simulink model "DFADAS2_SenFus_v1_201204RC_training_210115"  (R2018b)
settings: Solver=FixedStepDiscrete  StartTime=0.0  StopTime=inf  FixedStep=0.002  RelTol=1e-3  EnableMultiTasking=on
PreLoadFcn:
  | RTWConfigurationCB('preloadfcn', bdroot);
libraries: canmsglib x108, simulink x48, canfdmsglib x12
(part 13 of 28)

== system DFADAS2_SenFus_v1_201204RC_training_210115/Signal Input (Input)/Signal Input (50ms) (Input50)/Front Left Radar(S2) Objects Information (FLRdr)/S0 Data Frame Read/Subsystem ==
  Bus Creator : BusCreator  Inputs=10
  M0ObjInfo : Subsystem  TreatAsAtomicUnit=on
  M1ObjInfo1 : Subsystem  TreatAsAtomicUnit=on
  M2ObjInfo : Subsystem  TreatAsAtomicUnit=on
  M3ObjInfo : Subsystem  TreatAsAtomicUnit=on
  M4ObjInfo1 : Subsystem  TreatAsAtomicUnit=on
  RLRdrObjInfo : Outport
  wires:
  Bus Creator/1 -> RLRdrObjInfo/1  "RLRdrObjInfo"
  M1ObjInfo1/1(M10ObjInfo) -> Bus Creator/3  "M10ObjInfo"
  M3ObjInfo/1(M30ObjInfo) -> Bus Creator/7  "M30ObjInfo"
  M4ObjInfo1/1(M40ObjInfo) -> Bus Creator/9  "M40ObjInfo"
  M0ObjInfo/1(M00ObjInfo) -> Bus Creator/1  "M00ObjInfo"
  M2ObjInfo/1(M20ObjInfo) -> Bus Creator/5  "M20ObjInfo"
  M3ObjInfo/2(M31ObjInfo) -> Bus Creator/8  "M31ObjInfo"
  M0ObjInfo/2(M01ObjInfo) -> Bus Creator/2  "M01ObjInfo"
  M1ObjInfo1/2(M11ObjInfo) -> Bus Creator/4  "M11ObjInfo"
  M2ObjInfo/2(M21ObjInfo) -> Bus Creator/6  "M21ObjInfo"
  M4ObjInfo1/2(M41ObjInfo) -> Bus Creator/10  "M41ObjInfo"

== system DFADAS2_SenFus_v1_201204RC_training_210115/Signal Input (Input)/Signal Input (50ms) (Input50)/Front Left Radar(S2) Objects Information (FLRdr)/S0 Data Frame Read/VsblMnmt ==
  note: 虚拟帧的数据帧与Trailer帧的可见性管理逻辑
      | ——包括了对VFCnt回卷的考虑
  HFVFCnt : Inport
  LocVFCnt : Inport  Port=2
  Add : Sum  Inputs=+-
  Constant : Constant  Value=100
  Logical Operator : Logic  Operator=OR  AllPortsSameDT=off  OutDataTypeStr=boolean
  Relational Operator1 : RelationalOperator  OutDataTypeStr=boolean  RndMeth=Simplest
  Relational Operator2 : RelationalOperator  OutDataTypeStr=boolean  RndMeth=Simplest
  EnFlg : Outport
  wires:
  Add/1 -> Relational Operator2/1
  Constant/1 -> Relational Operator2/2
  Logical Operator/1 -> EnFlg/1
  Relational Operator2/1 -> Logical Operator/2
  HFVFCnt/1 -> Relational Operator1/1, Add/2
  Relational Operator1/1 -> Logical Operator/1
  LocVFCnt/1 -> Relational Operator1/2, Add/1

== system DFADAS2_SenFus_v1_201204RC_training_210115/Signal Input (Input)/Signal Input (50ms) (Input50)/Front Left Radar(S2) Objects Information (FLRdr)/S0 Header Frame Read/Enabled Subsystem ==
  note: Reset
  Msg : Inport
  Enable : EnablePort  StatesWhenEnabling=reset
  Bus Creator : BusCreator  Inputs=4
  CAN FD Unpack1 : canfdmsglib/CAN FD Unpack  CANdbFile=C:\Users\ThinkPad\Desktop\200529-海拉角雷达DBC\PR53671_DFPV_D53_HWA_SDE_F-SRR_CANFD_DF RESEARCH.dbc  MsgList=Object_Header_S2  MsgName=Object_Header_S2  ProtocolMode=CAN FD  MsgIDType=Standard (11-bit identifier)  MsgIdentifier=854  MsgLength=20  SignalInfo=NumberOfObjects_S2$67$5$1$2$1$0$1$0$0$30$#StateInfo_S2$0$3$1$2$1$0$1$0$0$7$#gPTPTimeStampOfData_HIGH_S2$35$32$1$2$1$0$1$0$0$4294967295$#gPTPTimeStampOfData_LOW_S2$3$32$1$2$1$0$1$0$0$4294967295$#  NSignals=4  IDPort=off  TimestampPort=off  ErrorPort=off  RemotePort=off  LengthPort=off  StatusPort=off  BRSPort=off  ESIPort=off  DLCPort=off  StartBits=str2num('[int32(67);int32(0);int32(35);int32(3)]')  SignalSizes=str2num('[int32(5);int32(3);int32(32);int32(32)]')  ByteOrders=str2num('[int32(1);int32(1);int32(1);int32(1)]')  DataTypes=str2num('[int32(2);int32(2);int32(2);int32(2)]')  MultiplexTypes=str2num('[int32(1);int32(1);int32(1);int32(1)]')  MultiplexValues=str2num('[double(0);double(0);double(0);double(0)]')  Factors=str2num('[double(1);double(1);double(1);double(1)]')  Offsets=str2num('[double(0);double(0);double(0);double(0)]')  Minimums=str2num('[double(0);double(0);double(0);double(0)]')  Maximums=str2num('[double(30);double(7);double(4294967295);double(4294967295)]')  ApplyMinMax=off
      settings: SourceProductName=Simulink Real-Time  DataFormat=manually specified signals
  Sigs : Outport
  wires:
  Msg/1 -> CAN FD Unpack1/1
  Bus Creator/1 -> Sigs/1  "FLRdr_bsCmnInfo"
  CAN FD Unpack1/1 -> Bus Creator/1  "NumberOfObjects_S2"
  CAN FD Unpack1/2 -> Bus Creator/2  "StateInfo_S2"
  CAN FD Unpack1/3 -> Bus Creator/3  "gPTPTimeStampOfData_LOW_S2"
  CAN FD Unpack1/4 -> Bus Creator/4  "gPTPTimeStampOfData_HIGH_S2"

== system DFADAS2_SenFus_v1_201204RC_training_210115/Signal Input (Input)/Signal Input (50ms) (Input50)/Front Left Radar(S2) Objects Information (FLRdr)/S0 Trailer Frame Read/VsblMnmt ==
  note: 虚拟帧的数据帧与Trailer帧的可见性管理逻辑
      | ——包括了对VFCnt回卷的考虑
  HFVFCnt : Inport
  LocVFCnt : Inport  Port=2
  Add : Sum  Inputs=+-
  Constant : Constant  Value=100
  Logical Operator : Logic  Operator=OR  AllPortsSameDT=off  OutDataTypeStr=boolean
  Relational Operator1 : RelationalOperator  OutDataTypeStr=boolean  RndMeth=Simplest
  Relational Operator2 : RelationalOperator  OutDataTypeStr=boolean  RndMeth=Simplest
  EnFlg : Outport
  wires:
  Add/1 -> Relational Operator2/1
  Constant/1 -> Relational Operator2/2
  Logical Operator/1 -> EnFlg/1
  Relational Operator2/1 -> Logical Operator/2
  HFVFCnt/1 -> Relational Operator1/1, Add/2
  Relational Operator1/1 -> Logical Operator/1
  LocVFCnt/1 -> Relational Operator1/2, Add/1

== system DFADAS2_SenFus_v1_201204RC_training_210115/Signal Input (Input)/Signal Input (50ms) (Input50)/Front Right Radar(S3) Objects Information (FRRdr)/S0 Data Frame Read/Enabled Subsystem ==
  note: Reset
  RemainderCnt : Inport
  Msg : Inport  Port=2
  obj_num : Inport  Port=3
  Enable : EnablePort  StatesWhenEnabling=reset
  Bus Creator : BusCreator  Inputs=10
  M0ObjInfo : Subsystem  TreatAsAtomicUnit=on
  M1ObjInfo1 : Subsystem  TreatAsAtomicUnit=on
  M2ObjInfo : Subsystem  TreatAsAtomicUnit=on
  M3ObjInfo : Subsystem  TreatAsAtomicUnit=on
  M4ObjInfo1 : Subsystem  TreatAsAtomicUnit=on
  Unpack : Subsystem
  RLRdrObjInfo : Outport
  wires:
  Msg/1 -> Unpack/1(Msg)
  Unpack/1(MsgOut) -> M0ObjInfo/1(msg), M4ObjInfo1/1(msg), M3ObjInfo/1(msg), M2ObjInfo/1(msg), M1ObjInfo1/1(msg)
  M0ObjInfo/1(M00ObjInfo) -> Bus Creator/1  "M00ObjInfo"
  M1ObjInfo1/1(M10ObjInfo) -> Bus Creator/3  "M10ObjInfo"
  M2ObjInfo/1(M20ObjInfo) -> Bus Creator/5  "M20ObjInfo"
  M3ObjInfo/1(M30ObjInfo) -> Bus Creator/7  "M30ObjInfo"
  M4ObjInfo1/1(M40ObjInfo) -> Bus Creator/9  "M40ObjInfo"
  Bus Creator/1 -> RLRdrObjInfo/1  "RLRdrObjInfo"
  RemainderCnt/1 -> Unpack/2(RemainderCnt), M0ObjInfo/3(RemainderCnt), M4ObjInfo1/3(RemainderCnt), M3ObjInfo/3(RemainderCnt), M2ObjInfo/3(RemainderCnt), M1ObjInfo1/3(RemainderCnt)
  Unpack/2(MValue) -> M4ObjInfo1/2(MValue), M3ObjInfo/2(MValue), M2ObjInfo/2(MValue), M1ObjInfo1/2(MValue), M0ObjInfo/2(MValue)
  M0ObjInfo/2(M01ObjInfo) -> Bus Creator/2  "M01ObjInfo"
  M1ObjInfo1/2(M11ObjInfo) -> Bus Creator/4  "M11ObjInfo"
  M2ObjInfo/2(M21ObjInfo) -> Bus Creator/6  "M21ObjInfo"
  M4ObjInfo1/2(M41ObjInfo) -> Bus Creator/10  "M41ObjInfo"
  M3ObjInfo/2(M31ObjInfo) -> Bus Creator/8  "M31ObjInfo"
  obj_num/1 -> M4ObjInfo1/4(obj_num), M3ObjInfo/4(obj_num), M2ObjInfo/4(obj_num), M1ObjInfo1/4(obj_num), M0ObjInfo/4(obj_num)

== system DFADAS2_SenFus_v1_201204RC_training_210115/Signal Input (Input)/Signal Input (50ms) (Input50)/Front Right Radar(S3) Objects Information (FRRdr)/S0 Data Frame Read/Subsystem ==
  Bus Creator : BusCreator  Inputs=10
  M0ObjInfo : Subsystem  TreatAsAtomicUnit=on
  M1ObjInfo1 : Subsystem  TreatAsAtomicUnit=on
  M2ObjInfo : Subsystem  TreatAsAtomicUnit=on
  M3ObjInfo : Subsystem  TreatAsAtomicUnit=on
  M4ObjInfo1 : Subsystem  TreatAsAtomicUnit=on
  RLRdrObjInfo : Outport
  wires:
  M4ObjInfo1/2(M41ObjInfo) -> Bus Creator/10  "M41ObjInfo"
  M2ObjInfo/2(M21ObjInfo) -> Bus Creator/6  "M21ObjInfo"
  M1ObjInfo1/2(M11ObjInfo) -> Bus Creator/4  "M11ObjInfo"
  M0ObjInfo/2(M01ObjInfo) -> Bus Creator/2  "M01ObjInfo"
  M3ObjInfo/2(M31ObjInfo) -> Bus Creator/8  "M31ObjInfo"
  M2ObjInfo/1(M20ObjInfo) -> Bus Creator/5  "M20ObjInfo"
  M0ObjInfo/1(M00ObjInfo) -> Bus Creator/1  "M00ObjInfo"
  M4ObjInfo1/1(M40ObjInfo) -> Bus Creator/9  "M40ObjInfo"
  M3ObjInfo/1(M30ObjInfo) -> Bus Creator/7  "M30ObjInfo"
  M1ObjInfo1/1(M10ObjInfo) -> Bus Creator/3  "M10ObjInfo"
  Bus Creator/1 -> RLRdrObjInfo/1  "RLRdrObjInfo"

== system DFADAS2_SenFus_v1_201204RC_training_210115/Signal Input (Input)/Signal Input (50ms) (Input50)/Front Right Radar(S3) Objects Information (FRRdr)/S0 Data Frame Read/VsblMnmt ==
  note: 虚拟帧的数据帧与Trailer帧的可见性管理逻辑
      | ——包括了对VFCnt回卷的考虑
  HFVFCnt : Inport
  LocVFCnt : Inport  Port=2
  Add : Sum  Inputs=+-
  Constant : Constant  Value=100
  Logical Operator : Logic  Operator=OR  AllPortsSameDT=off  OutDataTypeStr=boolean
  Relational Operator1 : RelationalOperator  OutDataTypeStr=boolean  RndMeth=Simplest
  Relational Operator2 : RelationalOperator  OutDataTypeStr=boolean  RndMeth=Simplest
  EnFlg : Outport
  wires:
  LocVFCnt/1 -> Add/1, Relational Operator1/2
  Relational Operator1/1 -> Logical Operator/1
  HFVFCnt/1 -> Add/2, Relational Operator1/1
  Relational Operator2/1 -> Logical Operator/2
  Logical Operator/1 -> EnFlg/1
  Constant/1 -> Relational Operator2/2
  Add/1 -> Relational Operator2/1

== system DFADAS2_SenFus_v1_201204RC_training_210115/Signal Input (Input)/Signal Input (50ms) (Input50)/Front Right Radar(S3) Objects Information (FRRdr)/S0 Header Frame Read/Enabled Subsystem ==
  note: Reset
  Msg : Inport
  Enable : EnablePort  StatesWhenEnabling=reset
  Bus Creator : BusCreator  Inputs=4
  CAN FD Unpack1 : canfdmsglib/CAN FD Unpack  CANdbFile=E:\200529-海拉角雷达DBC\PR53671_DFPV_D53_HWA_SDE_F-SRR_CANFD_DF RESEARCH.dbc  MsgList=Object_Header_S3  MsgName=Object_Header_S3  ProtocolMode=CAN FD  MsgIDType=Standard (11-bit identifier)  MsgIdentifier=857  MsgLength=20  SignalInfo=NumberOfObjects_S3$67$5$1$2$1$0$1$0$0$30$#StateInfo_S3$0$3$1$2$1$0$1$0$0$7$#gPTPTimeStampOfData_HIGH_S3$35$32$1$2$1$0$1$0$0$4294967295$#gPTPTimeStampOfData_LOW_S3$3$32$1$2$1$0$1$0$0$4294967295$#  NSignals=4  IDPort=off  TimestampPort=off  ErrorPort=off  RemotePort=off  LengthPort=off  StatusPort=off  BRSPort=off  ESIPort=off  DLCPort=off  StartBits=str2num('[int32(67);int32(0);int32(35);int32(3)]')  SignalSizes=str2num('[int32(5);int32(3);int32(32);int32(32)]')  ByteOrders=str2num('[int32(1);int32(1);int32(1);int32(1)]')  DataTypes=str2num('[int32(2);int32(2);int32(2);int32(2)]')  MultiplexTypes=str2num('[int32(1);int32(1);int32(1);int32(1)]')  MultiplexValues=str2num('[double(0);double(0);double(0);double(0)]')  Factors=str2num('[double(1);double(1);double(1);double(1)]')  Offsets=str2num('[double(0);double(0);double(0);double(0)]')  Minimums=str2num('[double(0);double(0);double(0);double(0)]')  Maximums=str2num('[double(30);double(7);double(4294967295);double(4294967295)]')  ApplyMinMax=off
      settings: SourceProductName=Simulink Real-Time  DataFormat=manually specified signals
  Sigs : Outport
  wires:
  Msg/1 -> CAN FD Unpack1/1
  Bus Creator/1 -> Sigs/1  "FRRdr_bsCmnInfo"
  CAN FD Unpack1/1 -> Bus Creator/1  "NumberOfObjects_S3"
  CAN FD Unpack1/2 -> Bus Creator/2  "StateInfo_S3"
  CAN FD Unpack1/3 -> Bus Creator/3  "gPTPTimeStampOfData_LOW_S3"
  CAN FD Unpack1/4 -> Bus Creator/4  "gPTPTimeStampOfData_HIGH_S3"

== system DFADAS2_SenFus_v1_201204RC_training_210115/Signal Input (Input)/Signal Input (50ms) (Input50)/Front Right Radar(S3) Objects Information (FRRdr)/S0 Trailer Frame Read/VsblMnmt ==
  note: 虚拟帧的数据帧与Trailer帧的可见性管理逻辑
      | ——包括了对VFCnt回卷的考虑
  HFVFCnt : Inport
  LocVFCnt : Inport  Port=2
  Add : Sum  Inputs=+-
  Constant : Constant  Value=100
  Logical Operator : Logic  Operator=OR  AllPortsSameDT=off  OutDataTypeStr=boolean
  Relational Operator1 : RelationalOperator  OutDataTypeStr=boolean  RndMeth=Simplest
  Relational Operator2 : RelationalOperator  OutDataTypeStr=boolean  RndMeth=Simplest
  EnFlg : Outport
  wires:
  LocVFCnt/1 -> Add/1, Relational Operator1/2
  Relational Operator1/1 -> Logical Operator/1
  HFVFCnt/1 -> Add/2, Relational Operator1/1
  Relational Operator2/1 -> Logical Operator/2
  Logical Operator/1 -> EnFlg/1
  Constant/1 -> Relational Operator2/2
  Add/1 -> Relational Operator2/1

== system DFADAS2_SenFus_v1_201204RC_training_210115/Signal Input (Input)/Signal Input (50ms) (Input50)/Rear Left Radar(S0) Objects Information (RLRdr)/S0 Data Frame Read/Enabled Subsystem ==
  note: Reset
  RemainderCnt : Inport
  Msg : Inport  Port=2
  obj_num : Inport  Port=3
  Enable : EnablePort  StatesWhenEnabling=reset
  Bus Creator : BusCreator  Inputs=10
  M0ObjInfo : Subsystem  TreatAsAtomicUnit=on
  M1ObjInfo1 : Subsystem  TreatAsAtomicUnit=on
  M2ObjInfo : Subsystem  TreatAsAtomicUnit=on
  M3ObjInfo : Subsystem  TreatAsAtomicUnit=on
  M4ObjInfo1 : Subsystem  TreatAsAtomicUnit=on
  Unpack : Subsystem
  RLRdrObjInfo : Outport
  wires:
  Msg/1 -> Unpack/1(Msg)
  Unpack/1(MsgOut) -> M0ObjInfo/1(msg), M4ObjInfo1/1(msg), M3ObjInfo/1(msg), M2ObjInfo/1(msg), M1ObjInfo1/1(msg)
  M0ObjInfo/1(M00ObjInfo) -> Bus Creator/1  "M00ObjInfo"
  M1ObjInfo1/1(M10ObjInfo) -> Bus Creator/3  "M10ObjInfo"
  M2ObjInfo/1(M20ObjInfo) -> Bus Creator/5  "M20ObjInfo"
  M3ObjInfo/1(M30ObjInfo) -> Bus Creator/7  "M30ObjInfo"
  M4ObjInfo1/1(M40ObjInfo) -> Bus Creator/9  "M40ObjInfo"
  Bus Creator/1 -> RLRdrObjInfo/1  "RLRdrObjInfo"
  RemainderCnt/1 -> Unpack/2(RemainderCnt), M0ObjInfo/3(RemainderCnt), M4ObjInfo1/3(RemainderCnt), M3ObjInfo/3(RemainderCnt), M2ObjInfo/3(RemainderCnt), M1ObjInfo1/3(RemainderCnt)
  Unpack/2(MValue) -> M4ObjInfo1/2(MValue), M3ObjInfo/2(MValue), M2ObjInfo/2(MValue), M1ObjInfo1/2(MValue), M0ObjInfo/2(MValue)
  M0ObjInfo/2(M01ObjInfo) -> Bus Creator/2  "M01ObjInfo"
  M1ObjInfo1/2(M11ObjInfo) -> Bus Creator/4  "M11ObjInfo"
  M2ObjInfo/2(M21ObjInfo) -> Bus Creator/6  "M21ObjInfo"
  M4ObjInfo1/2(M41ObjInfo) -> Bus Creator/10  "M41ObjInfo"
  M3ObjInfo/2(M31ObjInfo) -> Bus Creator/8  "M31ObjInfo"
  obj_num/1 -> M4ObjInfo1/4(obj_num), M3ObjInfo/4(obj_num), M2ObjInfo/4(obj_num), M1ObjInfo1/4(obj_num), M0ObjInfo/4(obj_num)

== system DFADAS2_SenFus_v1_201204RC_training_210115/Signal Input (Input)/Signal Input (50ms) (Input50)/Rear Left Radar(S0) Objects Information (RLRdr)/S0 Data Frame Read/Subsystem ==
  Bus Creator : BusCreator  Inputs=10
  M0ObjInfo : Subsystem  TreatAsAtomicUnit=on
  M1ObjInfo1 : Subsystem  TreatAsAtomicUnit=on
  M2ObjInfo : Subsystem  TreatAsAtomicUnit=on
  M3ObjInfo : Subsystem  TreatAsAtomicUnit=on
  M4ObjInfo1 : Subsystem  TreatAsAtomicUnit=on
  RLRdrObjInfo : Outport
  wires:
  M4ObjInfo1/2(M41ObjInfo) -> Bus Creator/10  "M41ObjInfo"
  M2ObjInfo/2(M21ObjInfo) -> Bus Creator/6  "M21ObjInfo"
  M1ObjInfo1/2(M11ObjInfo) -> Bus Creator/4  "M11ObjInfo"
  M0ObjInfo/2(M01ObjInfo) -> Bus Creator/2  "M01ObjInfo"
  M3ObjInfo/2(M31ObjInfo) -> Bus Creator/8  "M31ObjInfo"
  M2ObjInfo/1(M20ObjInfo) -> Bus Creator/5  "M20ObjInfo"
  M0ObjInfo/1(M00ObjInfo) -> Bus Creator/1  "M00ObjInfo"
  M4ObjInfo1/1(M40ObjInfo) -> Bus Creator/9  "M40ObjInfo"
  M3ObjInfo/1(M30ObjInfo) -> Bus Creator/7  "M30ObjInfo"
  M1ObjInfo1/1(M10ObjInfo) -> Bus Creator/3  "M10ObjInfo"
  Bus Creator/1 -> RLRdrObjInfo/1  "RLRdrObjInfo"

== system DFADAS2_SenFus_v1_201204RC_training_210115/Signal Input (Input)/Signal Input (50ms) (Input50)/Rear Left Radar(S0) Objects Information (RLRdr)/S0 Data Frame Read/VsblMnmt ==
  note: 虚拟帧的数据帧与Trailer帧的可见性管理逻辑
      | ——包括了对VFCnt回卷的考虑
  HFVFCnt : Inport
  LocVFCnt : Inport  Port=2
  Add : Sum  Inputs=+-
  Constant : Constant  Value=100
  Logical Operator : Logic  Operator=OR  AllPortsSameDT=off  OutDataTypeStr=boolean
  Relational Operator1 : RelationalOperator  OutDataTypeStr=boolean  RndMeth=Simplest
  Relational Operator2 : RelationalOperator  OutDataTypeStr=boolean  RndMeth=Simplest
  EnFlg : Outport
  wires:
  LocVFCnt/1 -> Add/1, Relational Operator1/2
  Relational Operator1/1 -> Logical Operator/1
  HFVFCnt/1 -> Add/2, Relational Operator1/1
  Relational Operator2/1 -> Logical Operator/2
  Logical Operator/1 -> EnFlg/1
  Constant/1 -> Relational Operator2/2
  Add/1 -> Relational Operator2/1

== system DFADAS2_SenFus_v1_201204RC_training_210115/Signal Input (Input)/Signal Input (50ms) (Input50)/Rear Left Radar(S0) Objects Information (RLRdr)/S0 Header Frame Read/Enabled Subsystem ==
  note: Reset
  Msg : Inport
  Enable : EnablePort  StatesWhenEnabling=reset
  Bus Creator : BusCreator  Inputs=4
  CAN FD Unpack1 : canfdmsglib/CAN FD Unpack  CANdbFile=D:\work\05_matlab\M18b\02_ACG18b_TC297woOS\04_DFCAN_test\PR53671_DFPV_D53_HWA_SDE_R-SRR_CANFD_DF_Research.dbc  MsgList=(none)  MsgName=Object_Header_S0  ProtocolMode=CAN FD  MsgIDType=Standard (11-bit identifier)  MsgIdentifier=848  MsgLength=20  SignalInfo=NumberOfObjects_S0$67$5$1$2$1$0$1$0$0$30$#StateInfo_S0$0$3$1$2$1$0$1$0$0$7$#gPTPTimeStampOfData_HIGH_S0$35$32$1$2$1$0$1$0$0$4294967295$#gPTPTimeStampOfData_LOW_S0$3$32$1$2$1$0$1$0$0$4294967295$#  NSignals=4  IDPort=off  TimestampPort=off  ErrorPort=off  RemotePort=off  LengthPort=off  StatusPort=off  BRSPort=off  ESIPort=off  DLCPort=off  StartBits=str2num('[int32(67);int32(0);int32(35);int32(3)]')  SignalSizes=str2num('[int32(5);int32(3);int32(32);int32(32)]')  ByteOrders=str2num('[int32(1);int32(1);int32(1);int32(1)]')  DataTypes=str2num('[int32(2);int32(2);int32(2);int32(2)]')  MultiplexTypes=str2num('[int32(1);int32(1);int32(1);int32(1)]')  MultiplexValues=str2num('[double(0);double(0);double(0);double(0)]')  Factors=str2num('[double(1);double(1);double(1);double(1)]')  Offsets=str2num('[double(0);double(0);double(0);double(0)]')  Minimums=str2num('[double(0);double(0);double(0);double(0)]')  Maximums=str2num('[double(30);double(7);double(4294967295);double(4294967295)]')  ApplyMinMax=off
      settings: SourceProductName=Simulink Real-Time  DataFormat=manually specified signals
  Sigs : Outport
  wires:
  Msg/1 -> CAN FD Unpack1/1
  Bus Creator/1 -> Sigs/1  "RLRdr_bsCmnInfo"
  CAN FD Unpack1/1 -> Bus Creator/1  "NumberOfObjects_S0"
  CAN FD Unpack1/2 -> Bus Creator/2  "StateInfo_S0"
  CAN FD Unpack1/3 -> Bus Creator/3  "gPTPTimeStampOfData_LOW_S0"
  CAN FD Unpack1/4 -> Bus Creator/4  "gPTPTimeStampOfData_HIGH_S0"

== system DFADAS2_SenFus_v1_201204RC_training_210115/Signal Input (Input)/Signal Input (50ms) (Input50)/Rear Left Radar(S0) Objects Information (RLRdr)/S0 Trailer Frame Read/VsblMnmt ==
  note: 虚拟帧的数据帧与Trailer帧的可见性管理逻辑
      | ——包括了对VFCnt回卷的考虑
  HFVFCnt : Inport
  LocVFCnt : Inport  Port=2
  Add : Sum  Inputs=+-
  Constant : Constant  Value=100
  Logical Operator : Logic  Operator=OR  AllPortsSameDT=off  OutDataTypeStr=boolean
  Relational Operator1 : RelationalOperator  OutDataTypeStr=boolean  RndMeth=Simplest
  Relational Operator2 : RelationalOperator  OutDataTypeStr=boolean  RndMeth=Simplest
  EnFlg : Outport
  wires:
  LocVFCnt/1 -> Add/1, Relational Operator1/2
  Relational Operator1/1 -> Logical Operator/1
  HFVFCnt/1 -> Add/2, Relational Operator1/1
  Relational Operator2/1 -> Logical Operator/2
  Logical Operator/1 -> EnFlg/1
  Constant/1 -> Relational Operator2/2
  Add/1 -> Relational Operator2/1

== system DFADAS2_SenFus_v1_201204RC_training_210115/Signal Input (Input)/Signal Input (50ms) (Input50)/Rear Right Radar(S1) Objects Information (RRRdr)/S0 Data Frame Read/Enabled Subsystem ==
  note: Reset
  RemainderCnt : Inport
  Msg : Inport  Port=2
  obj_num : Inport  Port=3
  Enable : EnablePort  StatesWhenEnabling=reset
  Bus Creator : BusCreator  Inputs=10
  M0ObjInfo : Subsystem  TreatAsAtomicUnit=on
  M1ObjInfo1 : Subsystem  TreatAsAtomicUnit=on
  M2ObjInfo : Subsystem  TreatAsAtomicUnit=on
  M3ObjInfo : Subsystem  TreatAsAtomicUnit=on
  M4ObjInfo1 : Subsystem  TreatAsAtomicUnit=on
  Unpack : Subsystem
  RLRdrObjInfo : Outport
  wires:
  obj_num/1 -> M0ObjInfo/4(obj_num), M1ObjInfo1/4(obj_num), M2ObjInfo/4(obj_num), M3ObjInfo/4(obj_num), M4ObjInfo1/4(obj_num)
  M3ObjInfo/2(M31ObjInfo) -> Bus Creator/8  "M31ObjInfo"
  M4ObjInfo1/2(M41ObjInfo) -> Bus Creator/10  "M41ObjInfo"
  M2ObjInfo/2(M21ObjInfo) -> Bus Creator/6  "M21ObjInfo"
  M1ObjInfo1/2(M11ObjInfo) -> Bus Creator/4  "M11ObjInfo"
  M0ObjInfo/2(M01ObjInfo) -> Bus Creator/2  "M01ObjInfo"
  Unpack/2(MValue) -> M0ObjInfo/2(MValue), M1ObjInfo1/2(MValue), M2ObjInfo/2(MValue), M3ObjInfo/2(MValue), M4ObjInfo1/2(MValue)
  RemainderCnt/1 -> M1ObjInfo1/3(RemainderCnt), M2ObjInfo/3(RemainderCnt), M3ObjInfo/3(RemainderCnt), M4ObjInfo1/3(RemainderCnt), M0ObjInfo/3(RemainderCnt), Unpack/2(RemainderCnt)
  Bus Creator/1 -> RLRdrObjInfo/1  "RLRdrObjInfo"
  M4ObjInfo1/1(M40ObjInfo) -> Bus Creator/9  "M40ObjInfo"
  M3ObjInfo/1(M30ObjInfo) -> Bus Creator/7  "M30ObjInfo"
  M2ObjInfo/1(M20ObjInfo) -> Bus Creator/5  "M20ObjInfo"
  M1ObjInfo1/1(M10ObjInfo) -> Bus Creator/3  "M10ObjInfo"
  M0ObjInfo/1(M00ObjInfo) -> Bus Creator/1  "M00ObjInfo"
  Unpack/1(MsgOut) -> M1ObjInfo1/1(msg), M2ObjInfo/1(msg), M3ObjInfo/1(msg), M4ObjInfo1/1(msg), M0ObjInfo/1(msg)
  Msg/1 -> Unpack/1(Msg)

== system DFADAS2_SenFus_v1_201204RC_training_210115/Signal Input (Input)/Signal Input (50ms) (Input50)/Rear Right Radar(S1) Objects Information (RRRdr)/S0 Data Frame Read/Subsystem ==
  Bus Creator : BusCreator  Inputs=10
  M0ObjInfo : Subsystem  TreatAsAtomicUnit=on
  M1ObjInfo1 : Subsystem  TreatAsAtomicUnit=on
  M2ObjInfo : Subsystem  TreatAsAtomicUnit=on
  M3ObjInfo : Subsystem  TreatAsAtomicUnit=on
  M4ObjInfo1 : Subsystem  TreatAsAtomicUnit=on
  RLRdrObjInfo : Outport
  wires:
  Bus Creator/1 -> RLRdrObjInfo/1  "RLRdrObjInfo"
  M1ObjInfo1/1(M10ObjInfo) -> Bus Creator/3  "M10ObjInfo"
  M3ObjInfo/1(M30ObjInfo) -> Bus Creator/7  "M30ObjInfo"
  M4ObjInfo1/1(M40ObjInfo) -> Bus Creator/9  "M40ObjInfo"
  M0ObjInfo/1(M00ObjInfo) -> Bus Creator/1  "M00ObjInfo"
  M2ObjInfo/1(M20ObjInfo) -> Bus Creator/5  "M20ObjInfo"
  M3ObjInfo/2(M31ObjInfo) -> Bus Creator/8  "M31ObjInfo"
  M0ObjInfo/2(M01ObjInfo) -> Bus Creator/2  "M01ObjInfo"
  M1ObjInfo1/2(M11ObjInfo) -> Bus Creator/4  "M11ObjInfo"
  M2ObjInfo/2(M21ObjInfo) -> Bus Creator/6  "M21ObjInfo"
  M4ObjInfo1/2(M41ObjInfo) -> Bus Creator/10  "M41ObjInfo"

== system DFADAS2_SenFus_v1_201204RC_training_210115/Signal Input (Input)/Signal Input (50ms) (Input50)/Rear Right Radar(S1) Objects Information (RRRdr)/S0 Data Frame Read/VsblMnmt ==
  note: 虚拟帧的数据帧与Trailer帧的可见性管理逻辑
      | ——包括了对VFCnt回卷的考虑
  HFVFCnt : Inport
  LocVFCnt : Inport  Port=2
  Add : Sum  Inputs=+-
  Constant : Constant  Value=100
  Logical Operator : Logic  Operator=OR  AllPortsSameDT=off  OutDataTypeStr=boolean
  Relational Operator1 : RelationalOperator  OutDataTypeStr=boolean  RndMeth=Simplest
  Relational Operator2 : RelationalOperator  OutDataTypeStr=boolean  RndMeth=Simplest
  EnFlg : Outport
  wires:
  Add/1 -> Relational Operator2/1
  Constant/1 -> Relational Operator2/2
  Logical Operator/1 -> EnFlg/1
  Relational Operator2/1 -> Logical Operator/2
  HFVFCnt/1 -> Relational Operator1/1, Add/2
  Relational Operator1/1 -> Logical Operator/1
  LocVFCnt/1 -> Relational Operator1/2, Add/1

== system DFADAS2_SenFus_v1_201204RC_training_210115/Signal Input (Input)/Signal Input (50ms) (Input50)/Rear Right Radar(S1) Objects Information (RRRdr)/S0 Header Frame Read/Enabled Subsystem ==
  note: Reset
  Msg : Inport
  Enable : EnablePort  StatesWhenEnabling=reset
  Bus Creator : BusCreator  Inputs=4
  CAN FD Unpack1 : canfdmsglib/CAN FD Unpack  CANdbFile=C:\Users\ThinkPad\Desktop\200529-海拉角雷达DBC\PR53671_DFPV_D53_HWA_SDE_F-SRR_CANFD_DF RESEARCH.dbc  MsgList=Object_Header_S1  MsgName=Object_Header_S1  ProtocolMode=CAN FD  MsgIDType=Standard (11-bit identifier)  MsgIdentifier=851  MsgLength=20  SignalInfo=NumberOfObjects_S1$67$5$1$2$1$0$1$0$0$30$#StateInfo_S1$0$3$1$2$1$0$1$0$0$7$#gPTPTimeStampOfData_HIGH_S1$35$32$1$2$1$0$1$0$0$4294967295$#gPTPTimeStampOfData_LOW_S1$3$32$1$2$1$0$1$0$0$4294967295$#  NSignals=4  IDPort=off  TimestampPort=off  ErrorPort=off  RemotePort=off  LengthPort=off  StatusPort=off  BRSPort=off  ESIPort=off  DLCPort=off  StartBits=str2num('[int32(67);int32(0);int32(35);int32(3)]')  SignalSizes=str2num('[int32(5);int32(3);int32(32);int32(32)]')  ByteOrders=str2num('[int32(1);int32(1);int32(1);int32(1)]')  DataTypes=str2num('[int32(2);int32(2);int32(2);int32(2)]')  MultiplexTypes=str2num('[int32(1);int32(1);int32(1);int32(1)]')  MultiplexValues=str2num('[double(0);double(0);double(0);double(0)]')  Factors=str2num('[double(1);double(1);double(1);double(1)]')  Offsets=str2num('[double(0);double(0);double(0);double(0)]')  Minimums=str2num('[double(0);double(0);double(0);double(0)]')  Maximums=str2num('[double(30);double(7);double(4294967295);double(4294967295)]')  ApplyMinMax=off
      settings: SourceProductName=Simulink Real-Time  DataFormat=manually specified signals
  Sigs : Outport
  wires:
  CAN FD Unpack1/3 -> Bus Creator/3  "gPTPTimeStampOfData_LOW_S1"
  CAN FD Unpack1/2 -> Bus Creator/2  "StateInfo_S1"
  CAN FD Unpack1/1 -> Bus Creator/1  "NumberOfObjects_S1"
  Bus Creator/1 -> Sigs/1  "RRRdr_bsCmnInfo"
  Msg/1 -> CAN FD Unpack1/1
  CAN FD Unpack1/4 -> Bus Creator/4  "gPTPTimeStampOfData_HIGH_S1"

== system DFADAS2_SenFus_v1_201204RC_training_210115/Signal Input (Input)/Signal Input (50ms) (Input50)/Rear Right Radar(S1) Objects Information (RRRdr)/S0 Trailer Frame Read/VsblMnmt ==
  note: 虚拟帧的数据帧与Trailer帧的可见性管理逻辑
      | ——包括了对VFCnt回卷的考虑
  HFVFCnt : Inport
  LocVFCnt : Inport  Port=2
  Add : Sum  Inputs=+-
  Constant : Constant  Value=100
  Logical Operator : Logic  Operator=OR  AllPortsSameDT=off  OutDataTypeStr=boolean
  Relational Operator1 : RelationalOperator  OutDataTypeStr=boolean  RndMeth=Simplest
  Relational Operator2 : RelationalOperator  OutDataTypeStr=boolean  RndMeth=Simplest
  EnFlg : Outport
  wires:
  Add/1 -> Relational Operator2/1
  Constant/1 -> Relational Operator2/2
  Logical Operator/1 -> EnFlg/1
  Relational Operator2/1 -> Logical Operator/2
  HFVFCnt/1 -> Relational Operator1/1, Add/2
  Relational Operator1/1 -> Logical Operator/1
  LocVFCnt/1 -> Relational Operator1/2, Add/1

== system DFADAS2_SenFus_v1_201204RC_training_210115/Signal Input (Input)/Signal Input (10ms) (Input10)/VehInfo/Body Electric System State Receive and Processing (BESRx)/Steering Lamp CAN Frame PreProcess (StLampCANFrmPPrcs)/CAN Diagnosis (CANDia) ==
  CANDia_tiCANRxSmplT : Inport
  CANDia_tiTLim : Inport  Port=2
  CANDia_cfNewFlg : Inport  Port=3
  CANDia_regCANMsg : Inport  Port=4
  CANDia_ctRllCnt : Inport  Port=5
  Break State Diagnosis (BreStDia) : Subsystem
  CAN Frame DTC Generator (CANFrmDTCGtr) : Subsystem
  CheckSum Diagnosis (ChkSumDia) : Subsystem
  RollingCounter Diagnosis (RllCntDia) : Subsystem
  wires:
  CANDia_regCANMsg/1 -> CheckSum Diagnosis (ChkSumDia)/1(ChkSumDia_regCANMsgPrev)
  CANDia_ctRllCnt/1 -> RollingCounter Diagnosis (RllCntDia)/1(RllCntChk_ctRollingCounter)
  RollingCounter Diagnosis (RllCntDia)/1(RllCntChk_efErrorFlag) -> CAN Frame DTC Generator (CANFrmDTCGtr)/3(CANFrmDTCGtr_efRllCntDiaErrFlg)
  Break State Diagnosis (BreStDia)/1(BreStDia_efErrFlg) -> CAN Frame DTC Generator (CANFrmDTCGtr)/1(CANFrmDTCGtr_efBreStDiaErrFlg)
  CheckSum Diagnosis (ChkSumDia)/1(ChkSumDia_efErrFlg) -> CAN Frame DTC Generator (CANFrmDTCGtr)/2(CANFrmDTCGtr_efChkSumDiaErrFlg)
  CANDia_cfNewFlg/1 -> Break State Diagnosis (BreStDia)/3(BreStDia_cfCANRxNewFlg)
  CANDia_tiTLim/1 -> Break State Diagnosis (BreStDia)/2(BreStDia_tiTLim)
  CANDia_tiCANRxSmplT/1 -> Break State Diagnosis (BreStDia)/1(BreStDia_tiCANRxSmplT)

== system DFADAS2_SenFus_v1_201204RC_training_210115/Signal Input (Input)/Signal Input (10ms) (Input10)/VehInfo/Function Keys State Receive and Processing (FKeyStRx)/Key Enable CAN Frame PreProcess (KeyEnaCANFrmPPrcs)/CAN Diagnosis (CANDia) ==
  CANDia_tiCANRxSmplT : Inport
  CANDia_tiTLim : Inport  Port=2
  CANDia_cfNewFlg : Inport  Port=3
  CANDia_regCANMsg : Inport  Port=4
  CANDia_ctRllCnt : Inport  Port=5
  Break State Diagnosis (BreStDia) : Subsystem
  CAN Frame DTC Generator (CANFrmDTCGtr) : Subsystem
  CheckSum Diagnosis (ChkSumDia) : Subsystem
  RollingCounter Diagnosis (RllCntDia) : Subsystem
  wires:
  CANDia_tiCANRxSmplT/1 -> Break State Diagnosis (BreStDia)/1(BreStDia_tiCANRxSmplT)
  CANDia_tiTLim/1 -> Break State Diagnosis (BreStDia)/2(BreStDia_tiTLim)
  CANDia_cfNewFlg/1 -> Break State Diagnosis (BreStDia)/3(BreStDia_cfCANRxNewFlg)
  CheckSum Diagnosis (ChkSumDia)/1(ChkSumDia_efErrFlg) -> CAN Frame DTC Generator (CANFrmDTCGtr)/2(CANFrmDTCGtr_efChkSumDiaErrFlg)
  Break State Diagnosis (BreStDia)/1(BreStDia_efErrFlg) -> CAN Frame DTC Generator (CANFrmDTCGtr)/1(CANFrmDTCGtr_efBreStDiaErrFlg)
  RollingCounter Diagnosis (RllCntDia)/1(RllCntChk_efErrorFlag) -> CAN Frame DTC Generator (CANFrmDTCGtr)/3(CANFrmDTCGtr_efRllCntDiaErrFlg)
  CANDia_ctRllCnt/1 -> RollingCounter Diagnosis (RllCntDia)/1(RllCntChk_ctRollingCounter)
  CANDia_regCANMsg/1 -> CheckSum Diagnosis (ChkSumDia)/1(ChkSumDia_regCANMsgPrev)

== system DFADAS2_SenFus_v1_201204RC_training_210115/Signal Input (Input)/Signal Input (10ms) (Input10)/VehInfo/MP5 Signal Receive (MP5Rx)1/CAN Diagnosis (CANDia)/Break State Diagnosis (BreStDia) ==
  note: Error Flag Discription:
      | 0 : Normal
      | 1 : Fault
  BreStDia_tiCANRxSmplT : Inport
  BreStDia_tiTLim : Inport  Port=2
  BreStDia_cfCANRxNewFlg : Inport  Port=3
  Add : Sum
  Add1 : Sum  Inputs=+-
  Constant : Constant  SampleTime=-1
  Constant1 : Constant  Value=0  SampleTime=-1
  Constant2 : Constant  Value=0  SampleTime=-1
  Constant3 : Constant  SampleTime=-1
  Divide : Product  Inputs=**
  Divide1 : Product  Inputs=/*
  Memory : Memory  InheritSampleTime=on
  Switch : Switch  Criteria=u2 ~= 0
  Switch1 : Switch
  BreStDia_efErrFlg : Outport
  wires:
  Constant1/1 -> Switch/1
  Constant/1 -> Switch/3
  Switch/1 -> Add/1, Divide/2
  Memory/1 -> Add/2
  Divide/1 -> Memory/1
  Add/1 -> Divide/1, Add1/2
  BreStDia_cfCANRxNewFlg/1 -> Switch/2
  BreStDia_tiCANRxSmplT/1 -> Divide1/1
  BreStDia_tiTLim/1 -> Divide1/2
  Add1/1 -> Switch1/2
  Constant2/1 -> Switch1/1
  Constant3/1 -> Switch1/3
  Switch1/1 -> BreStDia_efErrFlg/1
  Divide1/1 -> Add1/1

== system DFADAS2_SenFus_v1_201204RC_training_210115/Signal Input (Input)/Signal Input (10ms) (Input10)/VehInfo/MP5 Signal Receive (MP5Rx)1/CAN Diagnosis (CANDia)/CAN Frame DTC Generator (CANFrmDTCGtr) ==
  CANFrmDTCGtr_efBreStDiaErrFlg : Inport
  CANFrmDTCGtr_efChkSumDiaErrFlg : Inport  Port=2
  CANFrmDTCGtr_efRllCntDiaErrFlg : Inport  Port=3

== system DFADAS2_SenFus_v1_201204RC_training_210115/Signal Input (Input)/Signal Input (10ms) (Input10)/VehInfo/MP5 Signal Receive (MP5Rx)1/CAN Diagnosis (CANDia)/CheckSum Diagnosis (ChkSumDia) ==
  ChkSumDia_regCANMsgPrev : Inport
  Bit Check(BChk) : Subsystem  TreatAsAtomicUnit=on
      settings: RTWSystemCode=Nonreusable function
  CAN Message Data Extended (CMsgDaX) : S-Function  FunctionName=CANMsg_DataAcq  SFunctionDeploymentMode=off  EnableBusSupport=off  mask(CANMsg_DataExt){}
      mask help: This block extracts the raw data from the data field of the input CAN frame signal and outputs it as a 1-D array of data type uint8.
      mask Display:
      | color('blue');text(0.98,0.9,'NovSteeds','horizontalAlignment','right');color('black');text(0.5,0.5,'CAN Message\nData Extraction','horizontalAlignment','center');
      | port_label('input',1,'CAN_Msg');
      | port_label('output',1,'RawData');
  ChkSumDia_efErrFlg : Outport
  wires:
  Bit Check(BChk)/1(BChk_efErrFlg) -> ChkSumDia_efErrFlg/1
  ChkSumDia_regCANMsgPrev/1 -> CAN Message Data Extended (CMsgDaX)/1
  CAN Message Data Extended (CMsgDaX)/1 -> Bit Check(BChk)/1(BChk_bRawDa)

== system DFADAS2_SenFus_v1_201204RC_training_210115/Signal Input (Input)/Signal Input (10ms) (Input10)/VehInfo/MP5 Signal Receive (MP5Rx)1/CAN Diagnosis (CANDia)/RollingCounter Diagnosis (RllCntDia) ==
  note: RollingCounter Error Flag Discription:
      | 1 : Fault
      | 0 : Normal
  RllCntChk_ctRollingCounter : Inport
  Add : Sum  Inputs=+-
  Add1 : Sum  Inputs=+-
  Constant : Constant  OutDataTypeStr=single  SampleTime=-1
  Constant1 : Constant  Value=0  OutDataTypeStr=single  SampleTime=-1
  Constant2 : Constant  Value=-1  OutDataTypeStr=single  SampleTime=-1
  Constant3 : Constant  OutDataTypeStr=single  SampleTime=-1
  Data Type Conversion : DataTypeConversion  OutDataTypeStr=single
  Switch : Switch  Criteria=u2 ~= 0
  Switch1 : Switch  Threshold=14.5
  Unit Delay : UnitDelay  SampleTime=-1
  RllCntChk_efErrorFlag : Outport
  wires:
  RllCntChk_ctRollingCounter/1 -> Data Type Conversion/1
  Add/1 -> Add1/1
  Constant/1 -> Add1/2
  Constant1/1 -> Switch/3
  Constant3/1 -> Switch/1
  Add1/1 -> Switch/2
  Data Type Conversion/1 -> Add/1, Unit Delay/1
  Unit Delay/1 -> Switch1/2, Switch1/3
  Switch1/1 -> Add/2
  Constant2/1 -> Switch1/1
  Switch/1 -> RllCntChk_efErrorFlag/1

== system DFADAS2_SenFus_v1_201204RC_training_210115/Signal Input (Input)/Signal Input (10ms) (Input10)/VehInfo/Vehicle Movement Signal Receive and Processing (VehMovRx)/VehSpd CAN Frame PreProcess (VehSpdCANFrmPPrcs)/CAN Diagnosis (CANDia) ==
  CANDia_tiCANRxSmplT : Inport
  CANDia_tiTLim : Inport  Port=2
  CANDia_cfNewFlg : Inport  Port=3
  CANDia_regCANMsg : Inport  Port=4
  CANDia_ctRllCnt : Inport  Port=5
  Break State Diagnosis (BreStDia) : Subsystem
  CAN Frame DTC Generator (CANFrmDTCGtr) : Subsystem
  CheckSum Diagnosis (ChkSumDia) : Subsystem
  RollingCounter Diagnosis (RllCntDia) : Subsystem
  wires:
  CANDia_tiCANRxSmplT/1 -> Break State Diagnosis (BreStDia)/1(BreStDia_tiCANRxSmplT)
  CANDia_tiTLim/1 -> Break State Diagnosis (BreStDia)/2(BreStDia_tiTLim)
  CANDia_cfNewFlg/1 -> Break State Diagnosis (BreStDia)/3(BreStDia_cfCANRxNewFlg)
  CheckSum Diagnosis (ChkSumDia)/1(ChkSumDia_efErrFlg) -> CAN Frame DTC Generator (CANFrmDTCGtr)/2(CANFrmDTCGtr_efChkSumDiaErrFlg)
  Break State Diagnosis (BreStDia)/1(BreStDia_efErrFlg) -> CAN Frame DTC Generator (CANFrmDTCGtr)/1(CANFrmDTCGtr_efBreStDiaErrFlg)
  RollingCounter Diagnosis (RllCntDia)/1(RllCntChk_efErrorFlag) -> CAN Frame DTC Generator (CANFrmDTCGtr)/3(CANFrmDTCGtr_efRllCntDiaErrFlg)
  CANDia_ctRllCnt/1 -> RollingCounter Diagnosis (RllCntDia)/1(RllCntChk_ctRollingCounter)
  CANDia_regCANMsg/1 -> CheckSum Diagnosis (ChkSumDia)/1(ChkSumDia_regCANMsgPrev)

== system DFADAS2_SenFus_v1_201204RC_training_210115/Signal Input (Input)/Signal Input (10ms) (Input10)/VehInfo/Vehicle Movement Signal Receive and Processing (VehMovRx)/Yaw State CAN Frame PreProcess (YawCANFrmPPrcs)/CAN Diagnosis (CANDia) ==
  CANDia_tiCANRxSmplT : Inport
  CANDia_tiTLim : Inport  Port=2
  CANDia_cfNewFlg : Inport  Port=3
  CANDia_regCANMsg : Inport  Port=4
  CANDia_ctRllCnt : Inport  Port=5
  Break State Diagnosis (BreStDia) : Subsystem
  CAN Frame DTC Generator (CANFrmDTCGtr) : Subsystem
  CheckSum Diagnosis (ChkSumDia) : Subsystem
  RollingCounter Diagnosis (RllCntDia) : Subsystem
  wires:
  CANDia_tiCANRxSmplT/1 -> Break State Diagnosis (BreStDia)/1(BreStDia_tiCANRxSmplT)
  CANDia_tiTLim/1 -> Break State Diagnosis (BreStDia)/2(BreStDia_tiTLim)
  CANDia_cfNewFlg/1 -> Break State Diagnosis (BreStDia)/3(BreStDia_cfCANRxNewFlg)
  CheckSum Diagnosis (ChkSumDia)/1(ChkSumDia_efErrFlg) -> CAN Frame DTC Generator (CANFrmDTCGtr)/2(CANFrmDTCGtr_efChkSumDiaErrFlg)
  Break State Diagnosis (BreStDia)/1(BreStDia_efErrFlg) -> CAN Frame DTC Generator (CANFrmDTCGtr)/1(CANFrmDTCGtr_efBreStDiaErrFlg)
  RollingCounter Diagnosis (RllCntDia)/1(RllCntChk_efErrorFlag) -> CAN Frame DTC Generator (CANFrmDTCGtr)/3(CANFrmDTCGtr_efRllCntDiaErrFlg)
  CANDia_ctRllCnt/1 -> RollingCounter Diagnosis (RllCntDia)/1(RllCntChk_ctRollingCounter)
  CANDia_regCANMsg/1 -> CheckSum Diagnosis (ChkSumDia)/1(ChkSumDia_regCANMsgPrev)

== system DFADAS2_SenFus_v1_201204RC_training_210115/Signal Input (Input)/Signal Input (50ms) (Input50)/Cmr/CmrInfo/L0 Information (L0Info) /CAN Diagnosis (CANDia)1 ==
  CANDia_tiCANRxSmplT : Inport
  CANDia_tiTLim : Inport  Port=2
  CANDia_cfNewFlg : Inport  Port=3
  CANDia_regCANMsg : Inport  Port=4
  CANDia_ctRllCnt : Inport  Port=5
  Break State Diagnosis (BreStDia) : Subsystem
  CAN Frame DTC Generator (CANFrmDTCGtr) : Subsystem
  CheckSum Diagnosis (ChkSumDia) : Subsystem
  RollingCounter Diagnosis (RllCntDia) : Subsystem
  wires:
  CANDia_tiCANRxSmplT/1 -> Break State Diagnosis (BreStDia)/1(BreStDia_tiCANRxSmplT)
  CANDia_tiTLim/1 -> Break State Diagnosis (BreStDia)/2(BreStDia_tiTLim)
  CANDia_cfNewFlg/1 -> Break State Diagnosis (BreStDia)/3(BreStDia_cfCANRxNewFlg)
  CheckSum Diagnosis (ChkSumDia)/1(ChkSumDia_efErrFlg) -> CAN Frame DTC Generator (CANFrmDTCGtr)/2(CANFrmDTCGtr_efChkSumDiaErrFlg)
  Break State Diagnosis (BreStDia)/1(BreStDia_efErrFlg) -> CAN Frame DTC Generator (CANFrmDTCGtr)/1(CANFrmDTCGtr_efBreStDiaErrFlg)
  RollingCounter Diagnosis (RllCntDia)/1(RllCntChk_efErrorFlag) -> CAN Frame DTC Generator (CANFrmDTCGtr)/3(CANFrmDTCGtr_efRllCntDiaErrFlg)
  CANDia_ctRllCnt/1 -> RollingCounter Diagnosis (RllCntDia)/1(RllCntChk_ctRollingCounter)
  CANDia_regCANMsg/1 -> CheckSum Diagnosis (ChkSumDia)/1(ChkSumDia_regCANMsgPrev)

== system DFADAS2_SenFus_v1_201204RC_training_210115/Signal Input (Input)/Signal Input (50ms) (Input50)/Cmr/CmrInfo/L0 Information (L0Info) /L0 Information Fault Synthesis (L0FaultSyn)1 ==
  CANDia_tiCANRxSmplT : Inport
  CANDia_tiTLim : Inport  Port=2
  CANDia_cfNewFlg : Inport  Port=3
  CANDia_regCANMsg : Inport  Port=4
  CANDia_ctRllCnt : Inport  Port=5
  uint16 : Constant  Value=0  OutDataTypeStr=uint16
  L0FaultSyn_efL0FaultSyn : Outport
  wires:
  uint16/1 -> L0FaultSyn_efL0FaultSyn/1

== system DFADAS2_SenFus_v1_201204RC_training_210115/Signal Input (Input)/Signal Input (50ms) (Input50)/Cmr/CmrInfo/L1 Information (L1Info)/CAN Diagnosis (CANDia) ==
  CANDia_tiCANRxSmplT : Inport
  CANDia_tiTLim : Inport  Port=2
  CANDia_cfNewFlg : Inport  Port=3
  CANDia_regCANMsg : Inport  Port=4
  CANDia_ctRllCnt : Inport  Port=5
  Break State Diagnosis (BreStDia) : Subsystem
  CAN Frame DTC Generator (CANFrmDTCGtr) : Subsystem
  CheckSum Diagnosis (ChkSumDia) : Subsystem
  RollingCounter Diagnosis (RllCntDia) : Subsystem
  wires:
  CANDia_tiCANRxSmplT/1 -> Break State Diagnosis (BreStDia)/1(BreStDia_tiCANRxSmplT)
  CANDia_tiTLim/1 -> Break State Diagnosis (BreStDia)/2(BreStDia_tiTLim)
  CANDia_cfNewFlg/1 -> Break State Diagnosis (BreStDia)/3(BreStDia_cfCANRxNewFlg)
  CheckSum Diagnosis (ChkSumDia)/1(ChkSumDia_efErrFlg) -> CAN Frame DTC Generator (CANFrmDTCGtr)/2(CANFrmDTCGtr_efChkSumDiaErrFlg)
  Break State Diagnosis (BreStDia)/1(BreStDia_efErrFlg) -> CAN Frame DTC Generator (CANFrmDTCGtr)/1(CANFrmDTCGtr_efBreStDiaErrFlg)
  RollingCounter Diagnosis (RllCntDia)/1(RllCntChk_efErrorFlag) -> CAN Frame DTC Generator (CANFrmDTCGtr)/3(CANFrmDTCGtr_efRllCntDiaErrFlg)
  CANDia_ctRllCnt/1 -> RollingCounter Diagnosis (RllCntDia)/1(RllCntChk_ctRollingCounter)
  CANDia_regCANMsg/1 -> CheckSum Diagnosis (ChkSumDia)/1(ChkSumDia_regCANMsgPrev)

== system DFADAS2_SenFus_v1_201204RC_training_210115/Signal Input (Input)/Signal Input (50ms) (Input50)/Cmr/CmrInfo/L1 Information (L1Info)/L0 Information Fault Synthesis (L0FaultSyn) ==
  CANDia_tiCANRxSmplT : Inport
  CANDia_tiTLim : Inport  Port=2
  CANDia_cfNewFlg : Inport  Port=3
  CANDia_regCANMsg : Inport  Port=4
  CANDia_ctRllCnt : Inport  Port=5
  uint16 : Constant  Value=0  OutDataTypeStr=uint16
  L0FaultSyn_efL0FaultSyn : Outport
  wires:
  uint16/1 -> L0FaultSyn_efL0FaultSyn/1

== system DFADAS2_SenFus_v1_201204RC_training_210115/Signal Input (Input)/Signal Input (50ms) (Input50)/Cmr/CmrInfo/R0 Information (R0Info)/CAN Diagnosis (CANDia) ==
  CANDia_tiCANRxSmplT : Inport
  CANDia_tiTLim : Inport  Port=2
  CANDia_cfNewFlg : Inport  Port=3
  CANDia_regCANMsg : Inport  Port=4
  CANDia_ctRllCnt : Inport  Port=5
  Break State Diagnosis (BreStDia) : Subsystem
  CAN Frame DTC Generator (CANFrmDTCGtr) : Subsystem
  CheckSum Diagnosis (ChkSumDia) : Subsystem
  RollingCounter Diagnosis (RllCntDia) : Subsystem
  wires:
  CANDia_tiCANRxSmplT/1 -> Break State Diagnosis (BreStDia)/1(BreStDia_tiCANRxSmplT)
  CANDia_tiTLim/1 -> Break State Diagnosis (BreStDia)/2(BreStDia_tiTLim)
  CANDia_cfNewFlg/1 -> Break State Diagnosis (BreStDia)/3(BreStDia_cfCANRxNewFlg)
  CheckSum Diagnosis (ChkSumDia)/1(ChkSumDia_efErrFlg) -> CAN Frame DTC Generator (CANFrmDTCGtr)/2(CANFrmDTCGtr_efChkSumDiaErrFlg)
  Break State Diagnosis (BreStDia)/1(BreStDia_efErrFlg) -> CAN Frame DTC Generator (CANFrmDTCGtr)/1(CANFrmDTCGtr_efBreStDiaErrFlg)
  RollingCounter Diagnosis (RllCntDia)/1(RllCntChk_efErrorFlag) -> CAN Frame DTC Generator (CANFrmDTCGtr)/3(CANFrmDTCGtr_efRllCntDiaErrFlg)
  CANDia_ctRllCnt/1 -> RollingCounter Diagnosis (RllCntDia)/1(RllCntChk_ctRollingCounter)
  CANDia_regCANMsg/1 -> CheckSum Diagnosis (ChkSumDia)/1(ChkSumDia_regCANMsgPrev)

== system DFADAS2_SenFus_v1_201204RC_training_210115/Signal Input (Input)/Signal Input (50ms) (Input50)/Cmr/CmrInfo/R0 Information (R0Info)/R0 Information Fault Synthesis (R0FaultSyn) ==
  CANDia_tiCANRxSmplT : Inport
  CANDia_tiTLim : Inport  Port=2
  CANDia_cfNewFlg : Inport  Port=3
  CANDia_regCANMsg : Inport  Port=4
  CANDia_ctRllCnt : Inport  Port=5
  uint16 : Constant  Value=0  OutDataTypeStr=uint16
  R0FaultSyn_efL0FaultSyn : Outport
  wires:
  uint16/1 -> R0FaultSyn_efL0FaultSyn/1

== system DFADAS2_SenFus_v1_201204RC_training_210115/Signal Input (Input)/Signal Input (50ms) (Input50)/Cmr/CmrInfo/R1 Information (R1Info)/CAN Diagnosis (CANDia) ==
  CANDia_tiCANRxSmplT : Inport
  CANDia_tiTLim : Inport  Port=2
  CANDia_cfNewFlg : Inport  Port=3
  CANDia_regCANMsg : Inport  Port=4
  CANDia_ctRllCnt : Inport  Port=5
  Break State Diagnosis (BreStDia) : Subsystem
  CAN Frame DTC Generator (CANFrmDTCGtr) : Subsystem
  CheckSum Diagnosis (ChkSumDia) : Subsystem
  RollingCounter Diagnosis (RllCntDia) : Subsystem
  wires:
  CANDia_regCANMsg/1 -> CheckSum Diagnosis (ChkSumDia)/1(ChkSumDia_regCANMsgPrev)
  CANDia_ctRllCnt/1 -> RollingCounter Diagnosis (RllCntDia)/1(RllCntChk_ctRollingCounter)
  RollingCounter Diagnosis (RllCntDia)/1(RllCntChk_efErrorFlag) -> CAN Frame DTC Generator (CANFrmDTCGtr)/3(CANFrmDTCGtr_efRllCntDiaErrFlg)
  Break State Diagnosis (BreStDia)/1(BreStDia_efErrFlg) -> CAN Frame DTC Generator (CANFrmDTCGtr)/1(CANFrmDTCGtr_efBreStDiaErrFlg)
  CheckSum Diagnosis (ChkSumDia)/1(ChkSumDia_efErrFlg) -> CAN Frame DTC Generator (CANFrmDTCGtr)/2(CANFrmDTCGtr_efChkSumDiaErrFlg)
  CANDia_cfNewFlg/1 -> Break State Diagnosis (BreStDia)/3(BreStDia_cfCANRxNewFlg)
  CANDia_tiTLim/1 -> Break State Diagnosis (BreStDia)/2(BreStDia_tiTLim)
  CANDia_tiCANRxSmplT/1 -> Break State Diagnosis (BreStDia)/1(BreStDia_tiCANRxSmplT)

== system DFADAS2_SenFus_v1_201204RC_training_210115/Signal Input (Input)/Signal Input (50ms) (Input50)/Cmr/CmrInfo/R1 Information (R1Info)/R0 Information Fault Synthesis (R0FaultSyn) ==
  CANDia_tiCANRxSmplT : Inport
  CANDia_tiTLim : Inport  Port=2
  CANDia_cfNewFlg : Inport  Port=3
  CANDia_regCANMsg : Inport  Port=4
  CANDia_ctRllCnt : Inport  Port=5
  uint16 : Constant  Value=0  OutDataTypeStr=uint16
  R0FaultSyn_efL0FaultSyn : Outport
  wires:
  uint16/1 -> R0FaultSyn_efL0FaultSyn/1

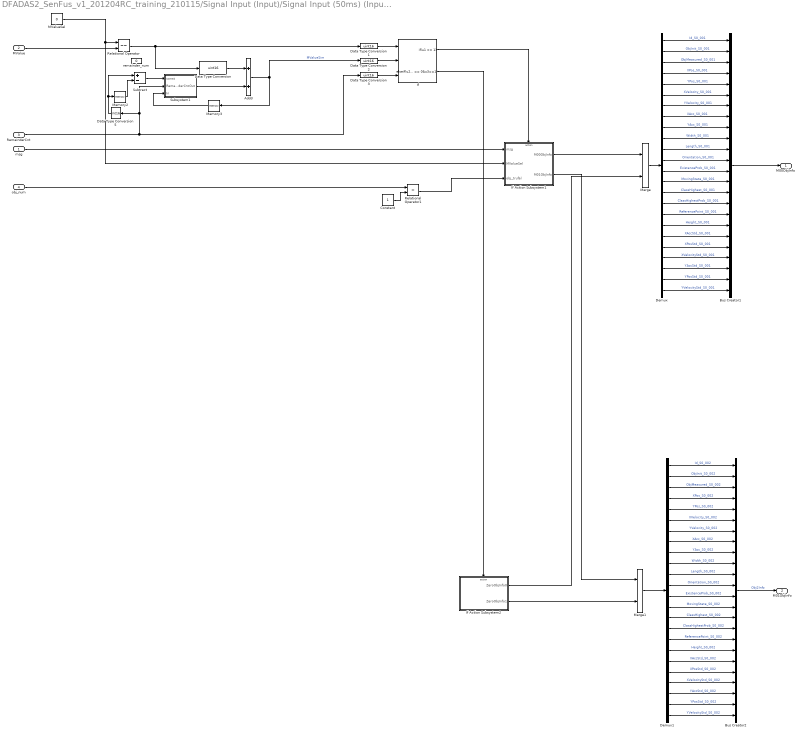
== system DFADAS2_SenFus_v1_201204RC_training_210115/Signal Input (Input)/Signal Input (50ms) (Input50)/Front Left Radar(S2) Objects Information (FLRdr)/S0 Data Frame Read/Enabled Subsystem/M0ObjInfo ==
  msg : Inport
  MValue : Inport  Port=2
  RemainderCnt : Inport  Port=3
  obj_num : Inport  Port=4
  Add3 : Sum
  Bus Creator1 : BusCreator  Inputs=24
  Bus Creator2 : BusCreator  Inputs=24
  Constant : Constant
  Data Type Conversion{,1..3} (4 alike) : DataTypeConversion  OutDataTypeStr=uint16
  Data Type Conversion5 : DataTypeConversion  OutDataTypeStr=int16
  Demux : Demux  Outputs=24
  Demux1 : Demux  Outputs=24
  If : If  NumInputs=3  IfExpression=u1 == 1  ElseIfExpressions=u2 == 0&u3==1  ShowElse=off
  If Action Subsystem1 : Subsystem  TreatAsAtomicUnit=on
  If Action Subsystem2 : Subsystem  TreatAsAtomicUnit=on
  MValueSel : Constant  Value=0
  Memory2 : Memory  InheritSampleTime=on
  Memory3 : Memory  InheritSampleTime=on
  Merge : Merge
  Merge1 : Merge
  Relational Operator : RelationalOperator  Operator===  OutDataTypeStr=boolean  RndMeth=Simplest
  Relational Operator1 : RelationalOperator  Operator=>  OutDataTypeStr=boolean  RndMeth=Simplest
  Subsystem1 : Subsystem
  Subtract : Sum  Inputs=+-
  remainder_num : Constant  Value=0  OutDataTypeStr=uint16
  M00ObjInfo : Outport
  M01ObjInfo : Outport  Port=2
  wires:
  Data Type Conversion5/1 -> Memory2/1, Subtract/1
  Memory3/1 -> Subsystem1/3(In)
  Subtract/1 -> Subsystem1/1(const)
  Memory2/1 -> Subtract/2
  Subsystem1/1(Out) -> Add3/2
  RemainderCnt/1 -> Data Type Conversion3/1, Subsystem1/2(RemainderCnt), Data Type Conversion5/1
  Data Type Conversion3/1 -> If/3
  Data Type Conversion2/1 -> If/2
  Data Type Conversion1/1 -> If/1
  Relational Operator1/1 -> If Action Subsystem1/3(obj_trufal)
  Constant/1 -> Relational Operator1/2
  obj_num/1 -> Relational Operator1/1
  Bus Creator2/1 -> M01ObjInfo/1  "Obj2Info"
  Merge1/1 -> Demux1/1
  Demux1/12 -> Bus Creator2/12  "Orientation_S0_002"
  Demux1/17 -> Bus Creator2/17  "ReferencePoint_S0_002"
  Demux1/22 -> Bus Creator2/22  "YAccStd_S0_002"
  Demux1/23 -> Bus Creator2/23  "YPosStd_S0_002"
  Demux1/8 -> Bus Creator2/8  "XAcc_S0_002"
  Demux1/21 -> Bus Creator2/21  "XVelocityStd_S0_002"
  Demux1/19 -> Bus Creator2/19  "XAccStd_S0_002"
  Demux1/18 -> Bus Creator2/18  "Height_S0_002"
  Demux1/15 -> Bus Creator2/15  "ClassHighest_S0_002"
  Demux1/7 -> Bus Creator2/7  "YVelocity_S0_002"
  Demux1/14 -> Bus Creator2/14  "MovingState_S0_002"
  Demux1/20 -> Bus Creator2/20  "XPosStd_S0_002"
  Demux1/13 -> Bus Creator2/13  "ExistenceProb_S0_002"
  Demux1/9 -> Bus Creator2/9  "YAcc_S0_002"
  Demux1/24 -> Bus Creator2/24  "YVelocityStd_S0_002"
  Demux1/11 -> Bus Creator2/11  "Length_S0_002"
  Demux1/10 -> Bus Creator2/10  "Width_S0_002"
  Demux1/4 -> Bus Creator2/4  "XPos_S0_002"
  Demux1/16 -> Bus Creator2/16  "ClassHighestProb_S0_002"
  Demux1/5 -> Bus Creator2/5  "YPos_S0_002"
  Demux1/3 -> Bus Creator2/3  "ObjMeasured_S0_002"
  Demux1/2 -> Bus Creator2/2  "ObjInit_S0_002"
  Demux1/6 -> Bus Creator2/6  "XVelocity_S0_002"
  Demux1/1 -> Bus Creator2/1  "Id_S0_002"
  Demux/6 -> Bus Creator1/6  "XVelocity_S0_001"
  Demux/1 -> Bus Creator1/1  "Id_S0_001"
  Demux/15 -> Bus Creator1/15  "ClassHighest_S0_001"
  Demux/11 -> Bus Creator1/11  "Length_S0_001"
  Demux/2 -> Bus Creator1/2  "ObjInit_S0_001"
  Demux/8 -> Bus Creator1/8  "XAcc_S0_001"
  Demux/19 -> Bus Creator1/19  "XAccStd_S0_001"
  Demux/4 -> Bus Creator1/4  "XPos_S0_001"
  Demux/21 -> Bus Creator1/21  "XVelocityStd_S0_001"
  Demux/16 -> Bus Creator1/16  "ClassHighestProb_S0_001"
  Demux/3 -> Bus Creator1/3  "ObjMeasured_S0_001"
  Demux/23 -> Bus Creator1/23  "YPosStd_S0_001"
  Demux/5 -> Bus Creator1/5  "YPos_S0_001"
  Demux/14 -> Bus Creator1/14  "MovingState_S0_001"
  Demux/9 -> Bus Creator1/9  "YAcc_S0_001"
  Demux/12 -> Bus Creator1/12  "Orientation_S0_001"
  Demux/18 -> Bus Creator1/18  "Height_S0_001"
  Demux/20 -> Bus Creator1/20  "XPosStd_S0_001"
  Demux/7 -> Bus Creator1/7  "YVelocity_S0_001"
  Demux/22 -> Bus Creator1/22  "YAccStd_S0_001"
  Demux/17 -> Bus Creator1/17  "ReferencePoint_S0_001"
  Demux/13 -> Bus Creator1/13  "ExistenceProb_S0_001"
  Demux/10 -> Bus Creator1/10  "Width_S0_001"
  Demux/24 -> Bus Creator1/24  "YVelocityStd_S0_001"
  Bus Creator1/1 -> M00ObjInfo/1
  Merge/1 -> Demux/1
  If Action Subsystem1/2(M01ObjInfo) -> Merge1/1
  If Action Subsystem2/2(ZeroObjInfo1) -> Merge1/2
  MValueSel/1 -> Relational Operator/1, If Action Subsystem1/2("MValueSel ")
  If Action Subsystem2/1(ZeroObjInfo0) -> Merge/2
  If Action Subsystem1/1(M00ObjInfo) -> Merge/1
  Relational Operator/1 -> Data Type Conversion1/1, Data Type Conversion/1
  If/2 -> If Action Subsystem2/Action
  If/1 -> If Action Subsystem1/Action
  Data Type Conversion/1 -> Add3/1
  Add3/1 -> Data Type Conversion2/1, Memory3/1  "MValueSim"
  MValue/1 -> Relational Operator/2
  msg/1 -> If Action Subsystem1/1(msg)
